simulink model "elevator"  (R2020a)
settings: Solver=VariableStepAuto  StartTime=0.0  StopTime=inf  RelTol=1e-3
PreLoadFcn:
  | slplc.api.loadDataTypes;
undefined symbols (not defined in the file): BOOL, DINT, INT, slplc
libraries: simulink x1
(part 24 of 38)

== system elevator/PLCControllerSuite/__Logic/Task/Program/__Logic/XIO6/RungInOverride ==
  In1 : Inport
  AND : Logic  AllPortsSameDT=off  OutDataTypeStr=boolean
  ForceRungInFalseRead : Subsystem  DisableCoverage=on  TreatAsAtomicUnit=on  mask{PLCLabelTag=_Force_RungIn_False, PLCBlockType=ForceRungInFalseRead}
      mask prompts: PLCLabelTag "Label Tag:"
      mask init:
      | block = gcb;
      | maskObj = Simulink.Mask.get(block);
      | maskObj.Display = sprintf('disp(''%s'');', PLCLabelTag);
      mask Help: web([docroot '/plccoder/ref/forcerunginfalseread' '.html']);
      mask DialogControl PLCBlockTitle Prompt: Force Rung-In False Read
      mask Display: disp('_Force_RungIn_False');
  NOT : Logic  Operator=NOT  IconShape=distinctive  AllPortsSameDT=off  OutDataTypeStr=boolean
  Out1 : Outport  VectorParamsAs1DForOutWhenUnconnected=off
  wires:
  AND/1 -> Out1/1
  In1/1 -> AND/2
  ForceRungInFalseRead/1(Out1) -> NOT/1
  NOT/1 -> AND/1

== system elevator/PLCControllerSuite/__Logic/Task/Program/__Logic/XIO6/__CoreVarRead ==
  DataRead : DataStoreRead  DataStoreName=xxx_PLC_VAR_AtFloor3
  y : Outport  VectorParamsAs1DForOutWhenUnconnected=off
  wires:
  DataRead/1 -> y/1

== system elevator/PLCControllerSuite/__Logic/Task/Program/__Logic/XIO7/BlockEnableRead ==
  __CoreLabelRead : Subsystem  Tag=CoreVarReadBlock  DisableCoverage=on  TreatAsAtomicUnit=on  mask{PLCBlockType=CoreLabelRead}
      mask init:
      | slplc.callbacks.initRoutineLabelRead(gcb);
      mask Help: web([docroot '/plccoder/ref/__corelabelread' '.html']);
      mask DialogControl PLCBlockTitle Prompt: Core Label Read
  Out1 : Outport  VectorParamsAs1DForOutWhenUnconnected=off
  wires:
  __CoreLabelRead/1(Out1) -> Out1/1

== system elevator/PLCControllerSuite/__Logic/Task/Program/__Logic/XIO7/Instruction_Enable ==
  Rung-condition-in : Inport  OutDataTypeStr=BOOL
  Enable : EnablePort
  Logical Operator : Logic  OutDataTypeStr=BOOL
  NOT : Logic  DisableCoverage=on  Operator=NOT  IconShape=distinctive  OutDataTypeStr=BOOL
  __CoreVarRead : Subsystem  Tag=CoreVarReadBlock  DisableCoverage=on  TreatAsAtomicUnit=on  mask{PLCBlockType=CoreVarRead}
      mask init:
      | slplc.callbacks.initCoreVariable(gcb, 'read');
      mask Help: web([docroot '/plccoder/ref/__corevarread' '.html']);
      mask DialogControl PLCBlockTitle Prompt: Core Variable Read
  Rung-condition-out : Outport  VectorParamsAs1DForOutWhenUnconnected=off
  wires:
  NOT/1 -> Logical Operator/2  "~DataBit"
  __CoreVarRead/1(y) -> NOT/1  "DataBit"
  Logical Operator/1 -> Rung-condition-out/1  "Rung-condition-out"
  Rung-condition-in/1 -> Logical Operator/1  "Rung-condition-in"

== system elevator/PLCControllerSuite/__Logic/Task/Program/__Logic/XIO7/RungInOverride ==
  In1 : Inport
  AND : Logic  AllPortsSameDT=off  OutDataTypeStr=boolean
  ForceRungInFalseRead : Subsystem  DisableCoverage=on  TreatAsAtomicUnit=on  mask{PLCLabelTag=_Force_RungIn_False, PLCBlockType=ForceRungInFalseRead}
      mask prompts: PLCLabelTag "Label Tag:"
      mask init:
      | block = gcb;
      | maskObj = Simulink.Mask.get(block);
      | maskObj.Display = sprintf('disp(''%s'');', PLCLabelTag);
      mask Help: web([docroot '/plccoder/ref/forcerunginfalseread' '.html']);
      mask DialogControl PLCBlockTitle Prompt: Force Rung-In False Read
      mask Display: disp('_Force_RungIn_False');
  NOT : Logic  Operator=NOT  IconShape=distinctive  AllPortsSameDT=off  OutDataTypeStr=boolean
  Out1 : Outport  VectorParamsAs1DForOutWhenUnconnected=off
  wires:
  NOT/1 -> AND/1
  ForceRungInFalseRead/1(Out1) -> NOT/1
  In1/1 -> AND/2
  AND/1 -> Out1/1

== system elevator/PLCControllerSuite/__Logic/Task/Program/__Logic/XIO7/__CoreVarRead ==
  DataRead : DataStoreRead  DataStoreName=xxx_PLC_VAR_AtFloor2
  y : Outport  VectorParamsAs1DForOutWhenUnconnected=off
  wires:
  DataRead/1 -> y/1

== system elevator/PLCControllerSuite/__Logic/Task/Program/__Logic/XIO8/BlockEnableRead ==
  __CoreLabelRead : Subsystem  Tag=CoreVarReadBlock  DisableCoverage=on  TreatAsAtomicUnit=on  mask{PLCBlockType=CoreLabelRead}
      mask init:
      | slplc.callbacks.initRoutineLabelRead(gcb);
      mask Help: web([docroot '/plccoder/ref/__corelabelread' '.html']);
      mask DialogControl PLCBlockTitle Prompt: Core Label Read
  Out1 : Outport  VectorParamsAs1DForOutWhenUnconnected=off
  wires:
  __CoreLabelRead/1(Out1) -> Out1/1

== system elevator/PLCControllerSuite/__Logic/Task/Program/__Logic/XIO8/Instruction_Enable ==
  Rung-condition-in : Inport  OutDataTypeStr=BOOL
  Enable : EnablePort
  Logical Operator : Logic  OutDataTypeStr=BOOL
  NOT : Logic  DisableCoverage=on  Operator=NOT  IconShape=distinctive  OutDataTypeStr=BOOL
  __CoreVarRead : Subsystem  Tag=CoreVarReadBlock  DisableCoverage=on  TreatAsAtomicUnit=on  mask{PLCBlockType=CoreVarRead}
      mask init:
      | slplc.callbacks.initCoreVariable(gcb, 'read');
      mask Help: web([docroot '/plccoder/ref/__corevarread' '.html']);
      mask DialogControl PLCBlockTitle Prompt: Core Variable Read
  Rung-condition-out : Outport  VectorParamsAs1DForOutWhenUnconnected=off
  wires:
  Rung-condition-in/1 -> Logical Operator/1  "Rung-condition-in"
  Logical Operator/1 -> Rung-condition-out/1  "Rung-condition-out"
  __CoreVarRead/1(y) -> NOT/1  "DataBit"
  NOT/1 -> Logical Operator/2  "~DataBit"

== system elevator/PLCControllerSuite/__Logic/Task/Program/__Logic/XIO8/RungInOverride ==
  In1 : Inport
  AND : Logic  AllPortsSameDT=off  OutDataTypeStr=boolean
  ForceRungInFalseRead : Subsystem  DisableCoverage=on  TreatAsAtomicUnit=on  mask{PLCLabelTag=_Force_RungIn_False, PLCBlockType=ForceRungInFalseRead}
      mask prompts: PLCLabelTag "Label Tag:"
      mask init:
      | block = gcb;
      | maskObj = Simulink.Mask.get(block);
      | maskObj.Display = sprintf('disp(''%s'');', PLCLabelTag);
      mask Help: web([docroot '/plccoder/ref/forcerunginfalseread' '.html']);
      mask DialogControl PLCBlockTitle Prompt: Force Rung-In False Read
      mask Display: disp('_Force_RungIn_False');
  NOT : Logic  Operator=NOT  IconShape=distinctive  AllPortsSameDT=off  OutDataTypeStr=boolean
  Out1 : Outport  VectorParamsAs1DForOutWhenUnconnected=off
  wires:
  AND/1 -> Out1/1
  In1/1 -> AND/2
  ForceRungInFalseRead/1(Out1) -> NOT/1
  NOT/1 -> AND/1

== system elevator/PLCControllerSuite/__Logic/Task/Program/__Logic/XIO8/__CoreVarRead ==
  DataRead : DataStoreRead  DataStoreName=xxx_PLC_VAR_AtFloor3
  y : Outport  VectorParamsAs1DForOutWhenUnconnected=off
  wires:
  DataRead/1 -> y/1

== system elevator/PLCControllerSuite/__Logic/Task/Program/__Logic/XIO9/BlockEnableRead ==
  __CoreLabelRead : Subsystem  Tag=CoreVarReadBlock  DisableCoverage=on  TreatAsAtomicUnit=on  mask{PLCBlockType=CoreLabelRead}
      mask init:
      | slplc.callbacks.initRoutineLabelRead(gcb);
      mask Help: web([docroot '/plccoder/ref/__corelabelread' '.html']);
      mask DialogControl PLCBlockTitle Prompt: Core Label Read
  Out1 : Outport  VectorParamsAs1DForOutWhenUnconnected=off
  wires:
  __CoreLabelRead/1(Out1) -> Out1/1

== system elevator/PLCControllerSuite/__Logic/Task/Program/__Logic/XIO9/Instruction_Enable ==
  Rung-condition-in : Inport  OutDataTypeStr=BOOL
  Enable : EnablePort
  Logical Operator : Logic  OutDataTypeStr=BOOL
  NOT : Logic  DisableCoverage=on  Operator=NOT  IconShape=distinctive  OutDataTypeStr=BOOL
  __CoreVarRead : Subsystem  Tag=CoreVarReadBlock  DisableCoverage=on  TreatAsAtomicUnit=on  mask{PLCBlockType=CoreVarRead}
      mask init:
      | slplc.callbacks.initCoreVariable(gcb, 'read');
      mask Help: web([docroot '/plccoder/ref/__corevarread' '.html']);
      mask DialogControl PLCBlockTitle Prompt: Core Variable Read
  Rung-condition-out : Outport  VectorParamsAs1DForOutWhenUnconnected=off
  wires:
  NOT/1 -> Logical Operator/2  "~DataBit"
  __CoreVarRead/1(y) -> NOT/1  "DataBit"
  Logical Operator/1 -> Rung-condition-out/1  "Rung-condition-out"
  Rung-condition-in/1 -> Logical Operator/1  "Rung-condition-in"

== system elevator/PLCControllerSuite/__Logic/Task/Program/__Logic/XIO9/RungInOverride ==
  In1 : Inport
  AND : Logic  AllPortsSameDT=off  OutDataTypeStr=boolean
  ForceRungInFalseRead : Subsystem  DisableCoverage=on  TreatAsAtomicUnit=on  mask{PLCLabelTag=_Force_RungIn_False, PLCBlockType=ForceRungInFalseRead}
      mask prompts: PLCLabelTag "Label Tag:"
      mask init:
      | block = gcb;
      | maskObj = Simulink.Mask.get(block);
      | maskObj.Display = sprintf('disp(''%s'');', PLCLabelTag);
      mask Help: web([docroot '/plccoder/ref/forcerunginfalseread' '.html']);
      mask DialogControl PLCBlockTitle Prompt: Force Rung-In False Read
      mask Display: disp('_Force_RungIn_False');
  NOT : Logic  Operator=NOT  IconShape=distinctive  AllPortsSameDT=off  OutDataTypeStr=boolean
  Out1 : Outport  VectorParamsAs1DForOutWhenUnconnected=off
  wires:
  NOT/1 -> AND/1
  ForceRungInFalseRead/1(Out1) -> NOT/1
  In1/1 -> AND/2
  AND/1 -> Out1/1

== system elevator/PLCControllerSuite/__Logic/Task/Program/__Logic/XIO9/__CoreVarRead ==
  DataRead : DataStoreRead  DataStoreName=xxx_PLC_VAR_AtFloor3
  y : Outport  VectorParamsAs1DForOutWhenUnconnected=off
  wires:
  DataRead/1 -> y/1

== system elevator/PLCControllerSuite/__Logic/Task/Program/__Logic/ADD/BlockEnableRead/__CoreLabelRead ==
  DataRead : DataStoreRead  DataStoreName=x_PLCLabel__s4_3653__Block_Enable
  Out1 : Outport  VectorParamsAs1DForOutWhenUnconnected=off
  wires:
  DataRead/1 -> Out1/1

== system elevator/PLCControllerSuite/__Logic/Task/Program/__Logic/ADD/RungInOverride/ForceRungInFalseRead ==
  __CoreLabelRead : Subsystem  Tag=CoreVarReadBlock  DisableCoverage=on  TreatAsAtomicUnit=on  mask{PLCBlockType=CoreLabelRead}
      mask init:
      | slplc.callbacks.initRoutineLabelRead(gcb);
      mask Help: web([docroot '/plccoder/ref/__corelabelread' '.html']);
      mask DialogControl PLCBlockTitle Prompt: Core Label Read
  Out1 : Outport  VectorParamsAs1DForOutWhenUnconnected=off
  wires:
  __CoreLabelRead/1(Out1) -> Out1/1

== system elevator/PLCControllerSuite/__Logic/Task/Program/__Logic/ADD/RungOutOverride/BlockEnableRead ==
  __CoreLabelRead : Subsystem  Tag=CoreVarReadBlock  DisableCoverage=on  TreatAsAtomicUnit=on  mask{PLCBlockType=CoreLabelRead}
      mask init:
      | slplc.callbacks.initRoutineLabelRead(gcb);
      mask Help: web([docroot '/plccoder/ref/__corelabelread' '.html']);
      mask DialogControl PLCBlockTitle Prompt: Core Label Read
  Out1 : Outport  VectorParamsAs1DForOutWhenUnconnected=off
  wires:
  __CoreLabelRead/1(Out1) -> Out1/1

== system elevator/PLCControllerSuite/__Logic/Task/Program/__Logic/ADD/RungOutOverride/VariableWriteEnableWrite ==
  In1 : Inport
  __CoreLabelWrite : Subsystem  Tag=CoreVarWriteBlock  DisableCoverage=on  TreatAsAtomicUnit=on  mask{PLCBlockType=CoreLabelWrite}
      mask init:
      | slplc.callbacks.initRoutineLabelWrite(gcb);
      mask Help: web([docroot '/plccoder/ref/__corelabelwrite' '.html']);
      mask DialogControl PLCBlockTitle Prompt: Core Label Write
  wires:
  In1/1 -> __CoreLabelWrite/1(In1)

== system elevator/PLCControllerSuite/__Logic/Task/Program/__Logic/EQU/BlockEnableRead/__CoreLabelRead ==
  DataRead : DataStoreRead  DataStoreName=x_PLCLabel__s4_3653__Block_Enable
  Out1 : Outport  VectorParamsAs1DForOutWhenUnconnected=off
  wires:
  DataRead/1 -> Out1/1

== system elevator/PLCControllerSuite/__Logic/Task/Program/__Logic/EQU/RungInOverride/ForceRungInFalseRead ==
  __CoreLabelRead : Subsystem  Tag=CoreVarReadBlock  DisableCoverage=on  TreatAsAtomicUnit=on  mask{PLCBlockType=CoreLabelRead}
      mask init:
      | slplc.callbacks.initRoutineLabelRead(gcb);
      mask Help: web([docroot '/plccoder/ref/__corelabelread' '.html']);
      mask DialogControl PLCBlockTitle Prompt: Core Label Read
  Out1 : Outport  VectorParamsAs1DForOutWhenUnconnected=off
  wires:
  __CoreLabelRead/1(Out1) -> Out1/1

== system elevator/PLCControllerSuite/__Logic/Task/Program/__Logic/EQU1/BlockEnableRead/__CoreLabelRead ==
  DataRead : DataStoreRead  DataStoreName=x_PLCLabel__s4_3653__Block_Enable
  Out1 : Outport  VectorParamsAs1DForOutWhenUnconnected=off
  wires:
  DataRead/1 -> Out1/1

== system elevator/PLCControllerSuite/__Logic/Task/Program/__Logic/EQU1/RungInOverride/ForceRungInFalseRead ==
  __CoreLabelRead : Subsystem  Tag=CoreVarReadBlock  DisableCoverage=on  TreatAsAtomicUnit=on  mask{PLCBlockType=CoreLabelRead}
      mask init:
      | slplc.callbacks.initRoutineLabelRead(gcb);
      mask Help: web([docroot '/plccoder/ref/__corelabelread' '.html']);
      mask DialogControl PLCBlockTitle Prompt: Core Label Read
  Out1 : Outport  VectorParamsAs1DForOutWhenUnconnected=off
  wires:
  __CoreLabelRead/1(Out1) -> Out1/1

== system elevator/PLCControllerSuite/__Logic/Task/Program/__Logic/EQU2/BlockEnableRead/__CoreLabelRead ==
  DataRead : DataStoreRead  DataStoreName=x_PLCLabel__s4_3653__Block_Enable
  Out1 : Outport  VectorParamsAs1DForOutWhenUnconnected=off
  wires:
  DataRead/1 -> Out1/1

== system elevator/PLCControllerSuite/__Logic/Task/Program/__Logic/EQU2/RungInOverride/ForceRungInFalseRead ==
  __CoreLabelRead : Subsystem  Tag=CoreVarReadBlock  DisableCoverage=on  TreatAsAtomicUnit=on  mask{PLCBlockType=CoreLabelRead}
      mask init:
      | slplc.callbacks.initRoutineLabelRead(gcb);
      mask Help: web([docroot '/plccoder/ref/__corelabelread' '.html']);
      mask DialogControl PLCBlockTitle Prompt: Core Label Read
  Out1 : Outport  VectorParamsAs1DForOutWhenUnconnected=off
  wires:
  __CoreLabelRead/1(Out1) -> Out1/1

== system elevator/PLCControllerSuite/__Logic/Task/Program/__Logic/EQU3/BlockEnableRead/__CoreLabelRead ==
  DataRead : DataStoreRead  DataStoreName=x_PLCLabel__s4_3653__Block_Enable
  Out1 : Outport  VectorParamsAs1DForOutWhenUnconnected=off
  wires:
  DataRead/1 -> Out1/1

== system elevator/PLCControllerSuite/__Logic/Task/Program/__Logic/EQU3/RungInOverride/ForceRungInFalseRead ==
  __CoreLabelRead : Subsystem  Tag=CoreVarReadBlock  DisableCoverage=on  TreatAsAtomicUnit=on  mask{PLCBlockType=CoreLabelRead}
      mask init:
      | slplc.callbacks.initRoutineLabelRead(gcb);
      mask Help: web([docroot '/plccoder/ref/__corelabelread' '.html']);
      mask DialogControl PLCBlockTitle Prompt: Core Label Read
  Out1 : Outport  VectorParamsAs1DForOutWhenUnconnected=off
  wires:
  __CoreLabelRead/1(Out1) -> Out1/1

== system elevator/PLCControllerSuite/__Logic/Task/Program/__Logic/GRT/BlockEnableRead/__CoreLabelRead ==
  DataRead : DataStoreRead  DataStoreName=x_PLCLabel__s4_3653__Block_Enable
  Out1 : Outport  VectorParamsAs1DForOutWhenUnconnected=off
  wires:
  DataRead/1 -> Out1/1

== system elevator/PLCControllerSuite/__Logic/Task/Program/__Logic/GRT/RungInOverride/ForceRungInFalseRead ==
  __CoreLabelRead : Subsystem  Tag=CoreVarReadBlock  DisableCoverage=on  TreatAsAtomicUnit=on  mask{PLCBlockType=CoreLabelRead}
      mask init:
      | slplc.callbacks.initRoutineLabelRead(gcb);
      mask Help: web([docroot '/plccoder/ref/__corelabelread' '.html']);
      mask DialogControl PLCBlockTitle Prompt: Core Label Read
  Out1 : Outport  VectorParamsAs1DForOutWhenUnconnected=off
  wires:
  __CoreLabelRead/1(Out1) -> Out1/1

== system elevator/PLCControllerSuite/__Logic/Task/Program/__Logic/Junction/BlockEnableRead/__CoreLabelRead ==
  DataRead : DataStoreRead  DataStoreName=x_PLCLabel__s4_3653__Block_Enable
  Out1 : Outport  VectorParamsAs1DForOutWhenUnconnected=off
  wires:
  DataRead/1 -> Out1/1

== system elevator/PLCControllerSuite/__Logic/Task/Program/__Logic/Junction1/BlockEnableRead/__CoreLabelRead ==
  DataRead : DataStoreRead  DataStoreName=x_PLCLabel__s4_3653__Block_Enable
  Out1 : Outport  VectorParamsAs1DForOutWhenUnconnected=off
  wires:
  DataRead/1 -> Out1/1

== system elevator/PLCControllerSuite/__Logic/Task/Program/__Logic/Junction10/BlockEnableRead/__CoreLabelRead ==
  DataRead : DataStoreRead  DataStoreName=x_PLCLabel__s4_3653__Block_Enable
  Out1 : Outport  VectorParamsAs1DForOutWhenUnconnected=off
  wires:
  DataRead/1 -> Out1/1

== system elevator/PLCControllerSuite/__Logic/Task/Program/__Logic/Junction11/BlockEnableRead/__CoreLabelRead ==
  DataRead : DataStoreRead  DataStoreName=x_PLCLabel__s4_3653__Block_Enable
  Out1 : Outport  VectorParamsAs1DForOutWhenUnconnected=off
  wires:
  DataRead/1 -> Out1/1

== system elevator/PLCControllerSuite/__Logic/Task/Program/__Logic/Junction12/BlockEnableRead/__CoreLabelRead ==
  DataRead : DataStoreRead  DataStoreName=x_PLCLabel__s4_3653__Block_Enable
  Out1 : Outport  VectorParamsAs1DForOutWhenUnconnected=off
  wires:
  DataRead/1 -> Out1/1

== system elevator/PLCControllerSuite/__Logic/Task/Program/__Logic/Junction13/BlockEnableRead/__CoreLabelRead ==
  DataRead : DataStoreRead  DataStoreName=x_PLCLabel__s4_3653__Block_Enable
  Out1 : Outport  VectorParamsAs1DForOutWhenUnconnected=off
  wires:
  DataRead/1 -> Out1/1

== system elevator/PLCControllerSuite/__Logic/Task/Program/__Logic/Junction14/BlockEnableRead/__CoreLabelRead ==
  DataRead : DataStoreRead  DataStoreName=x_PLCLabel__s4_3653__Block_Enable
  Out1 : Outport  VectorParamsAs1DForOutWhenUnconnected=off
  wires:
  DataRead/1 -> Out1/1

== system elevator/PLCControllerSuite/__Logic/Task/Program/__Logic/Junction15/BlockEnableRead/__CoreLabelRead ==
  DataRead : DataStoreRead  DataStoreName=x_PLCLabel__s4_3653__Block_Enable
  Out1 : Outport  VectorParamsAs1DForOutWhenUnconnected=off
  wires:
  DataRead/1 -> Out1/1

== system elevator/PLCControllerSuite/__Logic/Task/Program/__Logic/Junction16/BlockEnableRead/__CoreLabelRead ==
  DataRead : DataStoreRead  DataStoreName=x_PLCLabel__s4_3653__Block_Enable
  Out1 : Outport  VectorParamsAs1DForOutWhenUnconnected=off
  wires:
  DataRead/1 -> Out1/1

== system elevator/PLCControllerSuite/__Logic/Task/Program/__Logic/Junction17/BlockEnableRead/__CoreLabelRead ==
  DataRead : DataStoreRead  DataStoreName=x_PLCLabel__s4_3653__Block_Enable
  Out1 : Outport  VectorParamsAs1DForOutWhenUnconnected=off
  wires:
  DataRead/1 -> Out1/1

== system elevator/PLCControllerSuite/__Logic/Task/Program/__Logic/Junction18/BlockEnableRead/__CoreLabelRead ==
  DataRead : DataStoreRead  DataStoreName=x_PLCLabel__s4_3653__Block_Enable
  Out1 : Outport  VectorParamsAs1DForOutWhenUnconnected=off
  wires:
  DataRead/1 -> Out1/1

== system elevator/PLCControllerSuite/__Logic/Task/Program/__Logic/Junction19/BlockEnableRead/__CoreLabelRead ==
  DataRead : DataStoreRead  DataStoreName=x_PLCLabel__s4_3653__Block_Enable
  Out1 : Outport  VectorParamsAs1DForOutWhenUnconnected=off
  wires:
  DataRead/1 -> Out1/1

== system elevator/PLCControllerSuite/__Logic/Task/Program/__Logic/Junction2/BlockEnableRead/__CoreLabelRead ==
  DataRead : DataStoreRead  DataStoreName=x_PLCLabel__s4_3653__Block_Enable
  Out1 : Outport  VectorParamsAs1DForOutWhenUnconnected=off
  wires:
  DataRead/1 -> Out1/1

== system elevator/PLCControllerSuite/__Logic/Task/Program/__Logic/Junction20/BlockEnableRead/__CoreLabelRead ==
  DataRead : DataStoreRead  DataStoreName=x_PLCLabel__s4_3653__Block_Enable
  Out1 : Outport  VectorParamsAs1DForOutWhenUnconnected=off
  wires:
  DataRead/1 -> Out1/1

== system elevator/PLCControllerSuite/__Logic/Task/Program/__Logic/Junction21/BlockEnableRead/__CoreLabelRead ==
  DataRead : DataStoreRead  DataStoreName=x_PLCLabel__s4_3653__Block_Enable
  Out1 : Outport  VectorParamsAs1DForOutWhenUnconnected=off
  wires:
  DataRead/1 -> Out1/1

== system elevator/PLCControllerSuite/__Logic/Task/Program/__Logic/Junction22/BlockEnableRead/__CoreLabelRead ==
  DataRead : DataStoreRead  DataStoreName=x_PLCLabel__s4_3653__Block_Enable
  Out1 : Outport  VectorParamsAs1DForOutWhenUnconnected=off
  wires:
  DataRead/1 -> Out1/1

== system elevator/PLCControllerSuite/__Logic/Task/Program/__Logic/Junction23/BlockEnableRead/__CoreLabelRead ==
  DataRead : DataStoreRead  DataStoreName=x_PLCLabel__s4_3653__Block_Enable
  Out1 : Outport  VectorParamsAs1DForOutWhenUnconnected=off
  wires:
  DataRead/1 -> Out1/1

== system elevator/PLCControllerSuite/__Logic/Task/Program/__Logic/Junction24/BlockEnableRead/__CoreLabelRead ==
  DataRead : DataStoreRead  DataStoreName=x_PLCLabel__s4_3653__Block_Enable
  Out1 : Outport  VectorParamsAs1DForOutWhenUnconnected=off
  wires:
  DataRead/1 -> Out1/1

== system elevator/PLCControllerSuite/__Logic/Task/Program/__Logic/Junction25/BlockEnableRead/__CoreLabelRead ==
  DataRead : DataStoreRead  DataStoreName=x_PLCLabel__s4_3653__Block_Enable
  Out1 : Outport  VectorParamsAs1DForOutWhenUnconnected=off
  wires:
  DataRead/1 -> Out1/1

== system elevator/PLCControllerSuite/__Logic/Task/Program/__Logic/Junction26/BlockEnableRead/__CoreLabelRead ==
  DataRead : DataStoreRead  DataStoreName=x_PLCLabel__s4_3653__Block_Enable
  Out1 : Outport  VectorParamsAs1DForOutWhenUnconnected=off
  wires:
  DataRead/1 -> Out1/1

== system elevator/PLCControllerSuite/__Logic/Task/Program/__Logic/Junction27/BlockEnableRead/__CoreLabelRead ==
  DataRead : DataStoreRead  DataStoreName=x_PLCLabel__s4_3653__Block_Enable
  Out1 : Outport  VectorParamsAs1DForOutWhenUnconnected=off
  wires:
  DataRead/1 -> Out1/1

== system elevator/PLCControllerSuite/__Logic/Task/Program/__Logic/Junction28/BlockEnableRead/__CoreLabelRead ==
  DataRead : DataStoreRead  DataStoreName=x_PLCLabel__s4_3653__Block_Enable
  Out1 : Outport  VectorParamsAs1DForOutWhenUnconnected=off
  wires:
  DataRead/1 -> Out1/1

== system elevator/PLCControllerSuite/__Logic/Task/Program/__Logic/Junction29/BlockEnableRead/__CoreLabelRead ==
  DataRead : DataStoreRead  DataStoreName=x_PLCLabel__s4_3653__Block_Enable
  Out1 : Outport  VectorParamsAs1DForOutWhenUnconnected=off
  wires:
  DataRead/1 -> Out1/1

== system elevator/PLCControllerSuite/__Logic/Task/Program/__Logic/Junction3/BlockEnableRead/__CoreLabelRead ==
  DataRead : DataStoreRead  DataStoreName=x_PLCLabel__s4_3653__Block_Enable
  Out1 : Outport  VectorParamsAs1DForOutWhenUnconnected=off
  wires:
  DataRead/1 -> Out1/1

== system elevator/PLCControllerSuite/__Logic/Task/Program/__Logic/Junction30/BlockEnableRead/__CoreLabelRead ==
  DataRead : DataStoreRead  DataStoreName=x_PLCLabel__s4_3653__Block_Enable
  Out1 : Outport  VectorParamsAs1DForOutWhenUnconnected=off
  wires:
  DataRead/1 -> Out1/1

== system elevator/PLCControllerSuite/__Logic/Task/Program/__Logic/Junction31/BlockEnableRead/__CoreLabelRead ==
  DataRead : DataStoreRead  DataStoreName=x_PLCLabel__s4_3653__Block_Enable
  Out1 : Outport  VectorParamsAs1DForOutWhenUnconnected=off
  wires:
  DataRead/1 -> Out1/1

== system elevator/PLCControllerSuite/__Logic/Task/Program/__Logic/Junction32/BlockEnableRead/__CoreLabelRead ==
  DataRead : DataStoreRead  DataStoreName=x_PLCLabel__s4_3653__Block_Enable
  Out1 : Outport  VectorParamsAs1DForOutWhenUnconnected=off
  wires:
  DataRead/1 -> Out1/1

== system elevator/PLCControllerSuite/__Logic/Task/Program/__Logic/Junction33/BlockEnableRead/__CoreLabelRead ==
  DataRead : DataStoreRead  DataStoreName=x_PLCLabel__s4_3653__Block_Enable
  Out1 : Outport  VectorParamsAs1DForOutWhenUnconnected=off
  wires:
  DataRead/1 -> Out1/1

== system elevator/PLCControllerSuite/__Logic/Task/Program/__Logic/Junction34/BlockEnableRead/__CoreLabelRead ==
  DataRead : DataStoreRead  DataStoreName=x_PLCLabel__s4_3653__Block_Enable
  Out1 : Outport  VectorParamsAs1DForOutWhenUnconnected=off
  wires:
  DataRead/1 -> Out1/1

== system elevator/PLCControllerSuite/__Logic/Task/Program/__Logic/Junction35/BlockEnableRead/__CoreLabelRead ==
  DataRead : DataStoreRead  DataStoreName=x_PLCLabel__s4_3653__Block_Enable
  Out1 : Outport  VectorParamsAs1DForOutWhenUnconnected=off
  wires:
  DataRead/1 -> Out1/1

== system elevator/PLCControllerSuite/__Logic/Task/Program/__Logic/Junction4/BlockEnableRead/__CoreLabelRead ==
  DataRead : DataStoreRead  DataStoreName=x_PLCLabel__s4_3653__Block_Enable
  Out1 : Outport  VectorParamsAs1DForOutWhenUnconnected=off
  wires:
  DataRead/1 -> Out1/1

== system elevator/PLCControllerSuite/__Logic/Task/Program/__Logic/Junction5/BlockEnableRead/__CoreLabelRead ==
  DataRead : DataStoreRead  DataStoreName=x_PLCLabel__s4_3653__Block_Enable
  Out1 : Outport  VectorParamsAs1DForOutWhenUnconnected=off
  wires:
  DataRead/1 -> Out1/1

== system elevator/PLCControllerSuite/__Logic/Task/Program/__Logic/Junction6/BlockEnableRead/__CoreLabelRead ==
  DataRead : DataStoreRead  DataStoreName=x_PLCLabel__s4_3653__Block_Enable
  Out1 : Outport  VectorParamsAs1DForOutWhenUnconnected=off
  wires:
  DataRead/1 -> Out1/1

== system elevator/PLCControllerSuite/__Logic/Task/Program/__Logic/Junction7/BlockEnableRead/__CoreLabelRead ==
  DataRead : DataStoreRead  DataStoreName=x_PLCLabel__s4_3653__Block_Enable
  Out1 : Outport  VectorParamsAs1DForOutWhenUnconnected=off
  wires:
  DataRead/1 -> Out1/1

== system elevator/PLCControllerSuite/__Logic/Task/Program/__Logic/Junction8/BlockEnableRead/__CoreLabelRead ==
  DataRead : DataStoreRead  DataStoreName=x_PLCLabel__s4_3653__Block_Enable
  Out1 : Outport  VectorParamsAs1DForOutWhenUnconnected=off
  wires:
  DataRead/1 -> Out1/1

== system elevator/PLCControllerSuite/__Logic/Task/Program/__Logic/Junction9/BlockEnableRead/__CoreLabelRead ==
  DataRead : DataStoreRead  DataStoreName=x_PLCLabel__s4_3653__Block_Enable
  Out1 : Outport  VectorParamsAs1DForOutWhenUnconnected=off
  wires:
  DataRead/1 -> Out1/1

== system elevator/PLCControllerSuite/__Logic/Task/Program/__Logic/LEQ/BlockEnableRead/__CoreLabelRead ==
  DataRead : DataStoreRead  DataStoreName=x_PLCLabel__s4_3653__Block_Enable
  Out1 : Outport  VectorParamsAs1DForOutWhenUnconnected=off
  wires:
  DataRead/1 -> Out1/1

== system elevator/PLCControllerSuite/__Logic/Task/Program/__Logic/LEQ/RungInOverride/ForceRungInFalseRead ==
  __CoreLabelRead : Subsystem  Tag=CoreVarReadBlock  DisableCoverage=on  TreatAsAtomicUnit=on  mask{PLCBlockType=CoreLabelRead}
      mask init:
      | slplc.callbacks.initRoutineLabelRead(gcb);
      mask Help: web([docroot '/plccoder/ref/__corelabelread' '.html']);
      mask DialogControl PLCBlockTitle Prompt: Core Label Read
  Out1 : Outport  VectorParamsAs1DForOutWhenUnconnected=off
  wires:
  __CoreLabelRead/1(Out1) -> Out1/1

== system elevator/PLCControllerSuite/__Logic/Task/Program/__Logic/MOV/BlockEnableRead/__CoreLabelRead ==
  DataRead : DataStoreRead  DataStoreName=x_PLCLabel__s4_3653__Block_Enable
  Out1 : Outport  VectorParamsAs1DForOutWhenUnconnected=off
  wires:
  DataRead/1 -> Out1/1

== system elevator/PLCControllerSuite/__Logic/Task/Program/__Logic/MOV/RungInOverride/ForceRungInFalseRead ==
  __CoreLabelRead : Subsystem  Tag=CoreVarReadBlock  DisableCoverage=on  TreatAsAtomicUnit=on  mask{PLCBlockType=CoreLabelRead}
      mask init:
      | slplc.callbacks.initRoutineLabelRead(gcb);
      mask Help: web([docroot '/plccoder/ref/__corelabelread' '.html']);
      mask DialogControl PLCBlockTitle Prompt: Core Label Read
  Out1 : Outport  VectorParamsAs1DForOutWhenUnconnected=off
  wires:
  __CoreLabelRead/1(Out1) -> Out1/1

== system elevator/PLCControllerSuite/__Logic/Task/Program/__Logic/MOV/RungOutOverride/BlockEnableRead ==
  __CoreLabelRead : Subsystem  Tag=CoreVarReadBlock  DisableCoverage=on  TreatAsAtomicUnit=on  mask{PLCBlockType=CoreLabelRead}
      mask init:
      | slplc.callbacks.initRoutineLabelRead(gcb);
      mask Help: web([docroot '/plccoder/ref/__corelabelread' '.html']);
      mask DialogControl PLCBlockTitle Prompt: Core Label Read
  Out1 : Outport  VectorParamsAs1DForOutWhenUnconnected=off
  wires:
  __CoreLabelRead/1(Out1) -> Out1/1

== system elevator/PLCControllerSuite/__Logic/Task/Program/__Logic/MOV/RungOutOverride/VariableWriteEnableWrite ==
  In1 : Inport
  __CoreLabelWrite : Subsystem  Tag=CoreVarWriteBlock  DisableCoverage=on  TreatAsAtomicUnit=on  mask{PLCBlockType=CoreLabelWrite}
      mask init:
      | slplc.callbacks.initRoutineLabelWrite(gcb);
      mask Help: web([docroot '/plccoder/ref/__corelabelwrite' '.html']);
      mask DialogControl PLCBlockTitle Prompt: Core Label Write
  wires:
  In1/1 -> __CoreLabelWrite/1(In1)

== system elevator/PLCControllerSuite/__Logic/Task/Program/__Logic/MOV1/BlockEnableRead/__CoreLabelRead ==
  DataRead : DataStoreRead  DataStoreName=x_PLCLabel__s4_3653__Block_Enable
  Out1 : Outport  VectorParamsAs1DForOutWhenUnconnected=off
  wires:
  DataRead/1 -> Out1/1

== system elevator/PLCControllerSuite/__Logic/Task/Program/__Logic/MOV1/RungInOverride/ForceRungInFalseRead ==
  __CoreLabelRead : Subsystem  Tag=CoreVarReadBlock  DisableCoverage=on  TreatAsAtomicUnit=on  mask{PLCBlockType=CoreLabelRead}
      mask init:
      | slplc.callbacks.initRoutineLabelRead(gcb);
      mask Help: web([docroot '/plccoder/ref/__corelabelread' '.html']);
      mask DialogControl PLCBlockTitle Prompt: Core Label Read
  Out1 : Outport  VectorParamsAs1DForOutWhenUnconnected=off
  wires:
  __CoreLabelRead/1(Out1) -> Out1/1

== system elevator/PLCControllerSuite/__Logic/Task/Program/__Logic/MOV1/RungOutOverride/BlockEnableRead ==
  __CoreLabelRead : Subsystem  Tag=CoreVarReadBlock  DisableCoverage=on  TreatAsAtomicUnit=on  mask{PLCBlockType=CoreLabelRead}
      mask init:
      | slplc.callbacks.initRoutineLabelRead(gcb);
      mask Help: web([docroot '/plccoder/ref/__corelabelread' '.html']);
      mask DialogControl PLCBlockTitle Prompt: Core Label Read
  Out1 : Outport  VectorParamsAs1DForOutWhenUnconnected=off
  wires:
  __CoreLabelRead/1(Out1) -> Out1/1

== system elevator/PLCControllerSuite/__Logic/Task/Program/__Logic/MOV1/RungOutOverride/VariableWriteEnableWrite ==
  In1 : Inport
  __CoreLabelWrite : Subsystem  Tag=CoreVarWriteBlock  DisableCoverage=on  TreatAsAtomicUnit=on  mask{PLCBlockType=CoreLabelWrite}
      mask init:
      | slplc.callbacks.initRoutineLabelWrite(gcb);
      mask Help: web([docroot '/plccoder/ref/__corelabelwrite' '.html']);
      mask DialogControl PLCBlockTitle Prompt: Core Label Write
  wires:
  In1/1 -> __CoreLabelWrite/1(In1)

== system elevator/PLCControllerSuite/__Logic/Task/Program/__Logic/MOV2/BlockEnableRead/__CoreLabelRead ==
  DataRead : DataStoreRead  DataStoreName=x_PLCLabel__s4_3653__Block_Enable
  Out1 : Outport  VectorParamsAs1DForOutWhenUnconnected=off
  wires:
  DataRead/1 -> Out1/1

== system elevator/PLCControllerSuite/__Logic/Task/Program/__Logic/MOV2/RungInOverride/ForceRungInFalseRead ==
  __CoreLabelRead : Subsystem  Tag=CoreVarReadBlock  DisableCoverage=on  TreatAsAtomicUnit=on  mask{PLCBlockType=CoreLabelRead}
      mask init:
      | slplc.callbacks.initRoutineLabelRead(gcb);
      mask Help: web([docroot '/plccoder/ref/__corelabelread' '.html']);
      mask DialogControl PLCBlockTitle Prompt: Core Label Read
  Out1 : Outport  VectorParamsAs1DForOutWhenUnconnected=off
  wires:
  __CoreLabelRead/1(Out1) -> Out1/1

== system elevator/PLCControllerSuite/__Logic/Task/Program/__Logic/MOV2/RungOutOverride/BlockEnableRead ==
  __CoreLabelRead : Subsystem  Tag=CoreVarReadBlock  DisableCoverage=on  TreatAsAtomicUnit=on  mask{PLCBlockType=CoreLabelRead}
      mask init:
      | slplc.callbacks.initRoutineLabelRead(gcb);
      mask Help: web([docroot '/plccoder/ref/__corelabelread' '.html']);
      mask DialogControl PLCBlockTitle Prompt: Core Label Read
  Out1 : Outport  VectorParamsAs1DForOutWhenUnconnected=off
  wires:
  __CoreLabelRead/1(Out1) -> Out1/1

== system elevator/PLCControllerSuite/__Logic/Task/Program/__Logic/MOV2/RungOutOverride/VariableWriteEnableWrite ==
  In1 : Inport
  __CoreLabelWrite : Subsystem  Tag=CoreVarWriteBlock  DisableCoverage=on  TreatAsAtomicUnit=on  mask{PLCBlockType=CoreLabelWrite}
      mask init:
      | slplc.callbacks.initRoutineLabelWrite(gcb);
      mask Help: web([docroot '/plccoder/ref/__corelabelwrite' '.html']);
      mask DialogControl PLCBlockTitle Prompt: Core Label Write
  wires:
  In1/1 -> __CoreLabelWrite/1(In1)

== system elevator/PLCControllerSuite/__Logic/Task/Program/__Logic/MOV3/BlockEnableRead/__CoreLabelRead ==
  DataRead : DataStoreRead  DataStoreName=x_PLCLabel__s4_3653__Block_Enable
  Out1 : Outport  VectorParamsAs1DForOutWhenUnconnected=off
  wires:
  DataRead/1 -> Out1/1

== system elevator/PLCControllerSuite/__Logic/Task/Program/__Logic/MOV3/RungInOverride/ForceRungInFalseRead ==
  __CoreLabelRead : Subsystem  Tag=CoreVarReadBlock  DisableCoverage=on  TreatAsAtomicUnit=on  mask{PLCBlockType=CoreLabelRead}
      mask init:
      | slplc.callbacks.initRoutineLabelRead(gcb);
      mask Help: web([docroot '/plccoder/ref/__corelabelread' '.html']);
      mask DialogControl PLCBlockTitle Prompt: Core Label Read
  Out1 : Outport  VectorParamsAs1DForOutWhenUnconnected=off
  wires:
  __CoreLabelRead/1(Out1) -> Out1/1

== system elevator/PLCControllerSuite/__Logic/Task/Program/__Logic/MOV3/RungOutOverride/BlockEnableRead ==
  __CoreLabelRead : Subsystem  Tag=CoreVarReadBlock  DisableCoverage=on  TreatAsAtomicUnit=on  mask{PLCBlockType=CoreLabelRead}
      mask init:
      | slplc.callbacks.initRoutineLabelRead(gcb);
      mask Help: web([docroot '/plccoder/ref/__corelabelread' '.html']);
      mask DialogControl PLCBlockTitle Prompt: Core Label Read
  Out1 : Outport  VectorParamsAs1DForOutWhenUnconnected=off
  wires:
  __CoreLabelRead/1(Out1) -> Out1/1

== system elevator/PLCControllerSuite/__Logic/Task/Program/__Logic/MOV3/RungOutOverride/VariableWriteEnableWrite ==
  In1 : Inport
  __CoreLabelWrite : Subsystem  Tag=CoreVarWriteBlock  DisableCoverage=on  TreatAsAtomicUnit=on  mask{PLCBlockType=CoreLabelWrite}
      mask init:
      | slplc.callbacks.initRoutineLabelWrite(gcb);
      mask Help: web([docroot '/plccoder/ref/__corelabelwrite' '.html']);
      mask DialogControl PLCBlockTitle Prompt: Core Label Write
  wires:
  In1/1 -> __CoreLabelWrite/1(In1)

== system elevator/PLCControllerSuite/__Logic/Task/Program/__Logic/MOV4/BlockEnableRead/__CoreLabelRead ==
  DataRead : DataStoreRead  DataStoreName=x_PLCLabel__s4_3653__Block_Enable
  Out1 : Outport  VectorParamsAs1DForOutWhenUnconnected=off
  wires:
  DataRead/1 -> Out1/1

== system elevator/PLCControllerSuite/__Logic/Task/Program/__Logic/MOV4/RungInOverride/ForceRungInFalseRead ==
  __CoreLabelRead : Subsystem  Tag=CoreVarReadBlock  DisableCoverage=on  TreatAsAtomicUnit=on  mask{PLCBlockType=CoreLabelRead}
      mask init:
      | slplc.callbacks.initRoutineLabelRead(gcb);
      mask Help: web([docroot '/plccoder/ref/__corelabelread' '.html']);
      mask DialogControl PLCBlockTitle Prompt: Core Label Read
  Out1 : Outport  VectorParamsAs1DForOutWhenUnconnected=off
  wires:
  __CoreLabelRead/1(Out1) -> Out1/1

== system elevator/PLCControllerSuite/__Logic/Task/Program/__Logic/MOV4/RungOutOverride/BlockEnableRead ==
  __CoreLabelRead : Subsystem  Tag=CoreVarReadBlock  DisableCoverage=on  TreatAsAtomicUnit=on  mask{PLCBlockType=CoreLabelRead}
      mask init:
      | slplc.callbacks.initRoutineLabelRead(gcb);
      mask Help: web([docroot '/plccoder/ref/__corelabelread' '.html']);
      mask DialogControl PLCBlockTitle Prompt: Core Label Read
  Out1 : Outport  VectorParamsAs1DForOutWhenUnconnected=off
  wires:
  __CoreLabelRead/1(Out1) -> Out1/1

== system elevator/PLCControllerSuite/__Logic/Task/Program/__Logic/MOV4/RungOutOverride/VariableWriteEnableWrite ==
  In1 : Inport
  __CoreLabelWrite : Subsystem  Tag=CoreVarWriteBlock  DisableCoverage=on  TreatAsAtomicUnit=on  mask{PLCBlockType=CoreLabelWrite}
      mask init:
      | slplc.callbacks.initRoutineLabelWrite(gcb);
      mask Help: web([docroot '/plccoder/ref/__corelabelwrite' '.html']);
      mask DialogControl PLCBlockTitle Prompt: Core Label Write
  wires:
  In1/1 -> __CoreLabelWrite/1(In1)

== system elevator/PLCControllerSuite/__Logic/Task/Program/__Logic/MUL/BlockEnableRead/__CoreLabelRead ==
  DataRead : DataStoreRead  DataStoreName=x_PLCLabel__s4_3653__Block_Enable
  Out1 : Outport  VectorParamsAs1DForOutWhenUnconnected=off
  wires:
  DataRead/1 -> Out1/1

== system elevator/PLCControllerSuite/__Logic/Task/Program/__Logic/MUL/RungInOverride/ForceRungInFalseRead ==
  __CoreLabelRead : Subsystem  Tag=CoreVarReadBlock  DisableCoverage=on  TreatAsAtomicUnit=on  mask{PLCBlockType=CoreLabelRead}
      mask init:
      | slplc.callbacks.initRoutineLabelRead(gcb);
      mask Help: web([docroot '/plccoder/ref/__corelabelread' '.html']);
      mask DialogControl PLCBlockTitle Prompt: Core Label Read
  Out1 : Outport  VectorParamsAs1DForOutWhenUnconnected=off
  wires:
  __CoreLabelRead/1(Out1) -> Out1/1

== system elevator/PLCControllerSuite/__Logic/Task/Program/__Logic/MUL/RungOutOverride/BlockEnableRead ==
  __CoreLabelRead : Subsystem  Tag=CoreVarReadBlock  DisableCoverage=on  TreatAsAtomicUnit=on  mask{PLCBlockType=CoreLabelRead}
      mask init:
      | slplc.callbacks.initRoutineLabelRead(gcb);
      mask Help: web([docroot '/plccoder/ref/__corelabelread' '.html']);
      mask DialogControl PLCBlockTitle Prompt: Core Label Read
  Out1 : Outport  VectorParamsAs1DForOutWhenUnconnected=off
  wires:
  __CoreLabelRead/1(Out1) -> Out1/1

== system elevator/PLCControllerSuite/__Logic/Task/Program/__Logic/MUL/RungOutOverride/VariableWriteEnableWrite ==
  In1 : Inport
  __CoreLabelWrite : Subsystem  Tag=CoreVarWriteBlock  DisableCoverage=on  TreatAsAtomicUnit=on  mask{PLCBlockType=CoreLabelWrite}
      mask init:
      | slplc.callbacks.initRoutineLabelWrite(gcb);
      mask Help: web([docroot '/plccoder/ref/__corelabelwrite' '.html']);
      mask DialogControl PLCBlockTitle Prompt: Core Label Write
  wires:
  In1/1 -> __CoreLabelWrite/1(In1)

== system elevator/PLCControllerSuite/__Logic/Task/Program/__Logic/OTE/BlockEnableRead/__CoreLabelRead ==
  DataRead : DataStoreRead  DataStoreName=x_PLCLabel__s4_3653__Block_Enable
  Out1 : Outport  VectorParamsAs1DForOutWhenUnconnected=off
  wires:
  DataRead/1 -> Out1/1

== system elevator/PLCControllerSuite/__Logic/Task/Program/__Logic/OTE/Instruction_Enable/Initialize Function ==
  Constant : Constant  Value=0  OutDataTypeStr=BOOL
  Event Listener : EventListener  DisableCoverage=on  EventName=reset
  __CoreVarWrite : Subsystem  Tag=CoreVarWriteBlock  DisableCoverage=on  TreatAsAtomicUnit=on  mask{PLCBlockType=CoreVarWrite}
      mask init:
      | slplc.callbacks.initCoreVariable(gcb, 'write');
      mask Help: web([docroot '/plccoder/ref/__corevarwrite' '.html']);
      mask DialogControl PLCBlockTitle Prompt: Core Variable Write
  wires:
  Constant/1 -> __CoreVarWrite/1(u)

== system elevator/PLCControllerSuite/__Logic/Task/Program/__Logic/OTE/Instruction_Enable/Rung-condition is false ==
  Enable : EnablePort
  Constant : Constant  Value=0  OutDataTypeStr=BOOL
  __CoreVarWrite : Subsystem  Tag=CoreVarWriteBlock  DisableCoverage=on  TreatAsAtomicUnit=on  mask{PLCBlockType=CoreVarWrite}
      mask init:
      | slplc.callbacks.initCoreVariable(gcb, 'write');
      mask Help: web([docroot '/plccoder/ref/__corevarwrite' '.html']);
      mask DialogControl PLCBlockTitle Prompt: Core Variable Write
  wires:
  Constant/1 -> __CoreVarWrite/1(u)

== system elevator/PLCControllerSuite/__Logic/Task/Program/__Logic/OTE/Instruction_Enable/Rung-condition-in is true ==
  Enable : EnablePort
  Constant : Constant  OutDataTypeStr=BOOL
  __CoreVarWrite : Subsystem  Tag=CoreVarWriteBlock  DisableCoverage=on  TreatAsAtomicUnit=on  mask{PLCBlockType=CoreVarWrite}
      mask init:
      | slplc.callbacks.initCoreVariable(gcb, 'write');
      mask Help: web([docroot '/plccoder/ref/__corevarwrite' '.html']);
      mask DialogControl PLCBlockTitle Prompt: Core Variable Write
  wires:
  Constant/1 -> __CoreVarWrite/1(u)

== system elevator/PLCControllerSuite/__Logic/Task/Program/__Logic/OTE/RungInOverride/ForceRungInFalseRead ==
  __CoreLabelRead : Subsystem  Tag=CoreVarReadBlock  DisableCoverage=on  TreatAsAtomicUnit=on  mask{PLCBlockType=CoreLabelRead}
      mask init:
      | slplc.callbacks.initRoutineLabelRead(gcb);
      mask Help: web([docroot '/plccoder/ref/__corelabelread' '.html']);
      mask DialogControl PLCBlockTitle Prompt: Core Label Read
  Out1 : Outport  VectorParamsAs1DForOutWhenUnconnected=off
  wires:
  __CoreLabelRead/1(Out1) -> Out1/1

== system elevator/PLCControllerSuite/__Logic/Task/Program/__Logic/OTE1/BlockEnableRead/__CoreLabelRead ==
  DataRead : DataStoreRead  DataStoreName=x_PLCLabel__s4_3653__Block_Enable
  Out1 : Outport  VectorParamsAs1DForOutWhenUnconnected=off
  wires:
  DataRead/1 -> Out1/1

== system elevator/PLCControllerSuite/__Logic/Task/Program/__Logic/OTE1/Instruction_Enable/Initialize Function ==
  Constant : Constant  Value=0  OutDataTypeStr=BOOL
  Event Listener : EventListener  DisableCoverage=on  EventName=reset
  __CoreVarWrite : Subsystem  Tag=CoreVarWriteBlock  DisableCoverage=on  TreatAsAtomicUnit=on  mask{PLCBlockType=CoreVarWrite}
      mask init:
      | slplc.callbacks.initCoreVariable(gcb, 'write');
      mask Help: web([docroot '/plccoder/ref/__corevarwrite' '.html']);
      mask DialogControl PLCBlockTitle Prompt: Core Variable Write
  wires:
  Constant/1 -> __CoreVarWrite/1(u)

== system elevator/PLCControllerSuite/__Logic/Task/Program/__Logic/OTE1/Instruction_Enable/Rung-condition is false ==
  Enable : EnablePort
  Constant : Constant  Value=0  OutDataTypeStr=BOOL
  __CoreVarWrite : Subsystem  Tag=CoreVarWriteBlock  DisableCoverage=on  TreatAsAtomicUnit=on  mask{PLCBlockType=CoreVarWrite}
      mask init:
      | slplc.callbacks.initCoreVariable(gcb, 'write');
      mask Help: web([docroot '/plccoder/ref/__corevarwrite' '.html']);
      mask DialogControl PLCBlockTitle Prompt: Core Variable Write
  wires:
  Constant/1 -> __CoreVarWrite/1(u)

== system elevator/PLCControllerSuite/__Logic/Task/Program/__Logic/OTE1/Instruction_Enable/Rung-condition-in is true ==
  Enable : EnablePort
  Constant : Constant  OutDataTypeStr=BOOL
  __CoreVarWrite : Subsystem  Tag=CoreVarWriteBlock  DisableCoverage=on  TreatAsAtomicUnit=on  mask{PLCBlockType=CoreVarWrite}
      mask init:
      | slplc.callbacks.initCoreVariable(gcb, 'write');
      mask Help: web([docroot '/plccoder/ref/__corevarwrite' '.html']);
      mask DialogControl PLCBlockTitle Prompt: Core Variable Write
  wires:
  Constant/1 -> __CoreVarWrite/1(u)

== system elevator/PLCControllerSuite/__Logic/Task/Program/__Logic/OTE1/RungInOverride/ForceRungInFalseRead ==
  __CoreLabelRead : Subsystem  Tag=CoreVarReadBlock  DisableCoverage=on  TreatAsAtomicUnit=on  mask{PLCBlockType=CoreLabelRead}
      mask init:
      | slplc.callbacks.initRoutineLabelRead(gcb);
      mask Help: web([docroot '/plccoder/ref/__corelabelread' '.html']);
      mask DialogControl PLCBlockTitle Prompt: Core Label Read
  Out1 : Outport  VectorParamsAs1DForOutWhenUnconnected=off
  wires:
  __CoreLabelRead/1(Out1) -> Out1/1

== system elevator/PLCControllerSuite/__Logic/Task/Program/__Logic/OTE10/BlockEnableRead/__CoreLabelRead ==
  DataRead : DataStoreRead  DataStoreName=x_PLCLabel__s4_3653__Block_Enable
  Out1 : Outport  VectorParamsAs1DForOutWhenUnconnected=off
  wires:
  DataRead/1 -> Out1/1

== system elevator/PLCControllerSuite/__Logic/Task/Program/__Logic/OTE10/Instruction_Enable/Initialize Function ==
  Constant : Constant  Value=0  OutDataTypeStr=BOOL
  Event Listener : EventListener  DisableCoverage=on  EventName=reset
  __CoreVarWrite : Subsystem  Tag=CoreVarWriteBlock  DisableCoverage=on  TreatAsAtomicUnit=on  mask{PLCBlockType=CoreVarWrite}
      mask init:
      | slplc.callbacks.initCoreVariable(gcb, 'write');
      mask Help: web([docroot '/plccoder/ref/__corevarwrite' '.html']);
      mask DialogControl PLCBlockTitle Prompt: Core Variable Write
  wires:
  Constant/1 -> __CoreVarWrite/1(u)

== system elevator/PLCControllerSuite/__Logic/Task/Program/__Logic/OTE10/Instruction_Enable/Rung-condition is false ==
  Enable : EnablePort
  Constant : Constant  Value=0  OutDataTypeStr=BOOL
  __CoreVarWrite : Subsystem  Tag=CoreVarWriteBlock  DisableCoverage=on  TreatAsAtomicUnit=on  mask{PLCBlockType=CoreVarWrite}
      mask init:
      | slplc.callbacks.initCoreVariable(gcb, 'write');
      mask Help: web([docroot '/plccoder/ref/__corevarwrite' '.html']);
      mask DialogControl PLCBlockTitle Prompt: Core Variable Write
  wires:
  Constant/1 -> __CoreVarWrite/1(u)

== system elevator/PLCControllerSuite/__Logic/Task/Program/__Logic/OTE10/Instruction_Enable/Rung-condition-in is true ==
  Enable : EnablePort
  Constant : Constant  OutDataTypeStr=BOOL
  __CoreVarWrite : Subsystem  Tag=CoreVarWriteBlock  DisableCoverage=on  TreatAsAtomicUnit=on  mask{PLCBlockType=CoreVarWrite}
      mask init:
      | slplc.callbacks.initCoreVariable(gcb, 'write');
      mask Help: web([docroot '/plccoder/ref/__corevarwrite' '.html']);
      mask DialogControl PLCBlockTitle Prompt: Core Variable Write
  wires:
  Constant/1 -> __CoreVarWrite/1(u)

== system elevator/PLCControllerSuite/__Logic/Task/Program/__Logic/OTE10/RungInOverride/ForceRungInFalseRead ==
  __CoreLabelRead : Subsystem  Tag=CoreVarReadBlock  DisableCoverage=on  TreatAsAtomicUnit=on  mask{PLCBlockType=CoreLabelRead}
      mask init:
      | slplc.callbacks.initRoutineLabelRead(gcb);
      mask Help: web([docroot '/plccoder/ref/__corelabelread' '.html']);
      mask DialogControl PLCBlockTitle Prompt: Core Label Read
  Out1 : Outport  VectorParamsAs1DForOutWhenUnconnected=off
  wires:
  __CoreLabelRead/1(Out1) -> Out1/1

== system elevator/PLCControllerSuite/__Logic/Task/Program/__Logic/OTE11/BlockEnableRead/__CoreLabelRead ==
  DataRead : DataStoreRead  DataStoreName=x_PLCLabel__s4_3653__Block_Enable
  Out1 : Outport  VectorParamsAs1DForOutWhenUnconnected=off
  wires:
  DataRead/1 -> Out1/1

== system elevator/PLCControllerSuite/__Logic/Task/Program/__Logic/OTE11/Instruction_Enable/Initialize Function ==
  Constant : Constant  Value=0  OutDataTypeStr=BOOL
  Event Listener : EventListener  DisableCoverage=on  EventName=reset
  __CoreVarWrite : Subsystem  Tag=CoreVarWriteBlock  DisableCoverage=on  TreatAsAtomicUnit=on  mask{PLCBlockType=CoreVarWrite}
      mask init:
      | slplc.callbacks.initCoreVariable(gcb, 'write');
      mask Help: web([docroot '/plccoder/ref/__corevarwrite' '.html']);
      mask DialogControl PLCBlockTitle Prompt: Core Variable Write
  wires:
  Constant/1 -> __CoreVarWrite/1(u)

== system elevator/PLCControllerSuite/__Logic/Task/Program/__Logic/OTE11/Instruction_Enable/Rung-condition is false ==
  Enable : EnablePort
  Constant : Constant  Value=0  OutDataTypeStr=BOOL
  __CoreVarWrite : Subsystem  Tag=CoreVarWriteBlock  DisableCoverage=on  TreatAsAtomicUnit=on  mask{PLCBlockType=CoreVarWrite}
      mask init:
      | slplc.callbacks.initCoreVariable(gcb, 'write');
      mask Help: web([docroot '/plccoder/ref/__corevarwrite' '.html']);
      mask DialogControl PLCBlockTitle Prompt: Core Variable Write
  wires:
  Constant/1 -> __CoreVarWrite/1(u)

== system elevator/PLCControllerSuite/__Logic/Task/Program/__Logic/OTE11/Instruction_Enable/Rung-condition-in is true ==
  Enable : EnablePort
  Constant : Constant  OutDataTypeStr=BOOL
  __CoreVarWrite : Subsystem  Tag=CoreVarWriteBlock  DisableCoverage=on  TreatAsAtomicUnit=on  mask{PLCBlockType=CoreVarWrite}
      mask init:
      | slplc.callbacks.initCoreVariable(gcb, 'write');
      mask Help: web([docroot '/plccoder/ref/__corevarwrite' '.html']);
      mask DialogControl PLCBlockTitle Prompt: Core Variable Write
  wires:
  Constant/1 -> __CoreVarWrite/1(u)

== system elevator/PLCControllerSuite/__Logic/Task/Program/__Logic/OTE11/RungInOverride/ForceRungInFalseRead ==
  __CoreLabelRead : Subsystem  Tag=CoreVarReadBlock  DisableCoverage=on  TreatAsAtomicUnit=on  mask{PLCBlockType=CoreLabelRead}
      mask init:
      | slplc.callbacks.initRoutineLabelRead(gcb);
      mask Help: web([docroot '/plccoder/ref/__corelabelread' '.html']);
      mask DialogControl PLCBlockTitle Prompt: Core Label Read
  Out1 : Outport  VectorParamsAs1DForOutWhenUnconnected=off
  wires:
  __CoreLabelRead/1(Out1) -> Out1/1

== system elevator/PLCControllerSuite/__Logic/Task/Program/__Logic/OTE12/BlockEnableRead/__CoreLabelRead ==
  DataRead : DataStoreRead  DataStoreName=x_PLCLabel__s4_3653__Block_Enable
  Out1 : Outport  VectorParamsAs1DForOutWhenUnconnected=off
  wires:
  DataRead/1 -> Out1/1

== system elevator/PLCControllerSuite/__Logic/Task/Program/__Logic/OTE12/Instruction_Enable/Initialize Function ==
  Constant : Constant  Value=0  OutDataTypeStr=BOOL
  Event Listener : EventListener  DisableCoverage=on  EventName=reset
  __CoreVarWrite : Subsystem  Tag=CoreVarWriteBlock  DisableCoverage=on  TreatAsAtomicUnit=on  mask{PLCBlockType=CoreVarWrite}
      mask init:
      | slplc.callbacks.initCoreVariable(gcb, 'write');
      mask Help: web([docroot '/plccoder/ref/__corevarwrite' '.html']);
      mask DialogControl PLCBlockTitle Prompt: Core Variable Write
  wires:
  Constant/1 -> __CoreVarWrite/1(u)

== system elevator/PLCControllerSuite/__Logic/Task/Program/__Logic/OTE12/Instruction_Enable/Rung-condition is false ==
  Enable : EnablePort
  Constant : Constant  Value=0  OutDataTypeStr=BOOL
  __CoreVarWrite : Subsystem  Tag=CoreVarWriteBlock  DisableCoverage=on  TreatAsAtomicUnit=on  mask{PLCBlockType=CoreVarWrite}
      mask init:
      | slplc.callbacks.initCoreVariable(gcb, 'write');
      mask Help: web([docroot '/plccoder/ref/__corevarwrite' '.html']);
      mask DialogControl PLCBlockTitle Prompt: Core Variable Write
  wires:
  Constant/1 -> __CoreVarWrite/1(u)
